simulink model "p2"  (R2020b)
settings: Solver=VariableStepAuto  StartTime=0.0  StopTime=70  RelTol=1e-3
settings Model: Creator=Daniela  LastModifiedBy=Daniela

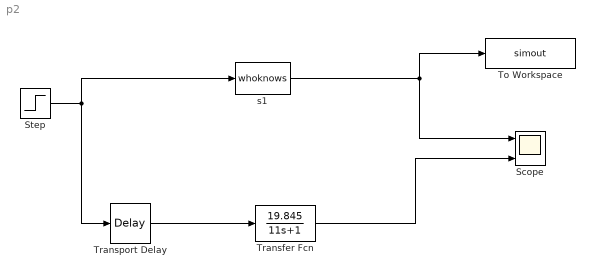
== system p2 ==
  Scope : Scope  NumInputPorts=3
  Step : Step  SampleTime=0
  To Workspace : ToWorkspace  VariableName=simout  SaveFormat=Timeseries  SampleTime=-1
  Transfer Fcn : TransferFcn  Numerator=[19.845]  Denominator=[11 1]
  Transport Delay : TransportDelay  DelayTime=3
  s1 : M-S-Function  FunctionName=whoknows  Parameters=L, P1, P2, T, R  mask{L=7, P1=0, P2=7, T=1, R=0}
      mask prompts: L "Laboratorio"; P1 "Primer digito del Puesto"; P2 "Segundo digito del Puesto"; T "Tipo de Planta"; R "Ruido"
      mask Display: disp('Sistema')
  wires:
  Step/1 -> s1/1, Transport Delay/1
  s1/1 -> To Workspace/1, Scope/1
  Transport Delay/1 -> Transfer Fcn/1
  Transfer Fcn/1 -> Scope/3
